simulink model "Control_try_final_2020b"  (R2020b)
settings: Solver=VariableStepAuto  StartTime=0.0  StopTime=inf  RelTol=1e-3
undefined symbols (not defined in the file or in its folder): DiscIntNeverNeededParam
libraries: mobileRoboticsLib x25
(part 6 of 7)

== stateflow chart Control_try_final_2020b/Team_1_behaviour/T1R2 (attacker 1)/Team 1 Behaviour1/kick_direction1/Chart2 ==
  state y_pos
    du:
    Vy = 1
  state y_neg
    du:
    Vy = -1
  (default) -> y_pos
  y_pos -> y_neg : [y > 0]
  y_neg -> y_pos : [y<1]
  data: y input; Vy output

== matlab function Control_try_final_2020b/Team_1_behaviour/T1R2 (attacker 1)/Team 1 Behaviour1/min_Distance_Finder/MATLAB Function ==
  data: min input; y output; rob3 input
function y = fcn(min, rob3)
 if min == rob3
y = 3;
 else 
     y =4;
 end
end

== stateflow chart Control_try_final_2020b/Team_1_behaviour/T1R2 (attacker 1)/Team 1 Behaviour1/min_Distance_Finder/R2_O_dist_val/Chart ==
  state calculate
    en:
    dist = 0;
    pos_x = 0;
    pos_y =0;
    dist_x =0;
    dist_y = 0;
    i=0;
    du:
    dist = 0;
    for i=1:7
    if (sen_1_val(i,3) > 4)
    pos_x = R_1_loc(1) + sen_1_val(i,1);
    pos_y = R_1_loc(2) + sen_1_val(i,2);
    dist_x = R_2_loc(1) - pos_x;
    dist_y = R_2_loc(2) - pos_y;
    dist = dist + sqrt((dist_x*dist_x) + (dist_y*dist_y));
    end
    end
  (default) -> calculate
  data: R_1_loc input; sen_1_val input; dist output; R_2_loc input; dist_y local; i local; pos_x local; pos_y local; dist_x local

== stateflow chart Control_try_final_2020b/Team_1_behaviour/T1R2 (attacker 1)/Team 1 Behaviour1/min_Distance_Finder/R3_O_dist_val/Chart ==
  state calculate
    en:
    dist = 0;
    pos_x = 0;
    pos_y =0;
    dist_x =0;
    dist_y = 0;
    i=0;
    du:
    dist = 0;
    for i=1:7
    if (sen_1_val(i,3) > 4)
    pos_x = R_1_loc(1) + sen_1_val(i,1);
    pos_y = R_1_loc(2) + sen_1_val(i,2);
    dist_x = R_2_loc(1) - pos_x;
    dist_y = R_2_loc(2) - pos_y;
    dist = dist + sqrt((dist_x*dist_x) + (dist_y*dist_y));
    end
    end
  (default) -> calculate
  data: R_1_loc input; sen_1_val input; dist output; R_2_loc input; dist_y local; i local; pos_x local; pos_y local; dist_x local

== stateflow chart Control_try_final_2020b/Team_1_behaviour/T1R2 (attacker 1)/Team 1 Behaviour1/min_Distance_Finder/R4_O_dist_val/Chart ==
  state calculate
    en:
    dist = 0;
    pos_x = 0;
    pos_y =0;
    dist_x =0;
    dist_y = 0;
    i=0;
    du:
    dist = 0;
    for i=1:7
    if (sen_1_val(i,3) > 4)
    pos_x = R_1_loc(1) + sen_1_val(i,1);
    pos_y = R_1_loc(2) + sen_1_val(i,2);
    dist_x = R_2_loc(1) - pos_x;
    dist_y = R_2_loc(2) - pos_y;
    dist = dist + sqrt((dist_x*dist_x) + (dist_y*dist_y));
    end
    end
  (default) -> calculate
  data: R_1_loc input; sen_1_val input; dist output; R_2_loc input; dist_y local; i local; pos_x local; pos_y local; dist_x local

== matlab function Control_try_final_2020b/Team_1_behaviour/T1R2 (attacker 1)/Team 1 Behaviour1/min_Distance_Finder/zero_padding ==
  data: u input; y output
function y = pad(u)
% Zero-pads object detections to work with arrays of buses

y = zeros(7,3);
numElems = min(size(u,1),7);
for idx = 1:numElems
   y(idx,1:3) = u(idx,1:3); 
end
end

== matlab function Control_try_final_2020b/Team_1_behaviour/T1R2 (attacker 1)/Team 1 Behaviour1/MATLAB Function3 ==
  data: distance_to_goal1 input; centroid output; goal_keeperY input; distance_to_goal2 input
function centroid  = shooting_spot_rev1_controller(distance_to_goal1, goal_keeperY, distance_to_goal2)
%UNTITLED3 Summary of this function goes here
%   Detailed explanation goes here
ShootingSpotFuzzyFile= getFISCodeGenerationData('shooting_spot_rev1');
C = evalfis(ShootingSpotFuzzyFile,[distance_to_goal1, goal_keeperY, distance_to_goal2]);
if ( C<1 )
% shooting_region=1;
centroid = [10,4.65];
elseif ( 1<=C && C<2 )
% shooting_region=2;
centroid = [10,3.35];
elseif ( 2<=C && C<3 )
% shooting_region=3;
centroid = [10,4.65];
else
% shooting_region=4;
centroid = [10,4.65];
end
end

== matlab function Control_try_final_2020b/Team_1_behaviour/T1R2 (attacker 1)/Team 1 Behaviour1/MATLAB Function2 ==
  data: u input; y output; r3 input; r4 input
function y = fcn(u , r3, r4)
if u == 3
   y = [r3(1), r3(2)];
else
    y = [r4(1) , r4(2)];
end

== matlab function Control_try_final_2020b/Team_1_behaviour/T1R2 (attacker 1)/Team 1 Behaviour1/MATLAB Function4 ==
  data: u input; y output
function y = fcn(u)
if u == 3
    y =1;
else 
    y = 0;
end
end

== matlab function Control_try_final_2020b/Team_1_behaviour/T1R3 (Defender 2)/Team 1 Behaviour1/MATLAB Function3 ==
  data: distance_to_goal1 input; centroid output; goal_keeperY input; distance_to_goal2 input
function centroid  = shooting_spot_rev1_controller(distance_to_goal1, goal_keeperY, distance_to_goal2)
%UNTITLED3 Summary of this function goes here
%   Detailed explanation goes here
ShootingSpotFuzzyFile= getFISCodeGenerationData('shooting_spot_rev1');
C = evalfis(ShootingSpotFuzzyFile,[distance_to_goal1, goal_keeperY, distance_to_goal2]);
if ( C<1 )
% shooting_region=1;
centroid = [10,4.65];
elseif ( 1<=C && C<2 )
% shooting_region=2;
centroid = [10,3.35];
elseif ( 2<=C && C<3 )
% shooting_region=3;
centroid = [10,4.65];
else
% shooting_region=4;
centroid = [10,4.65];
end
end

== matlab function Control_try_final_2020b/Team_1_behaviour/T1R3 (Defender 2)/Team 1 Behaviour1/MATLAB Function4 ==
  data: u input; y output
function y = fcn(u)
if u == 3
    y =1;
else 
    y = 0;
end
end

== stateflow chart Control_try_final_2020b/Team_1_behaviour/T1R3 (Defender 2)/Team 1 Behaviour1/kick_direction1/Chart1 ==
  state x_pos
    du:
    Vx = 1
  state x_neg
    du:
    Vx = -1
  (default) -> x_pos
  x_pos -> x_neg : [x > 0]
  x_neg -> x_pos : [x<1]
  data: Vx output; x input

== stateflow chart Control_try_final_2020b/Team_1_behaviour/T1R3 (Defender 2)/Team 1 Behaviour1/kick_direction1/Chart2 ==
  state y_pos
    du:
    Vy = 1
  state y_neg
    du:
    Vy = -1
  (default) -> y_pos
  y_pos -> y_neg : [y > 0]
  y_neg -> y_pos : [y<1]
  data: y input; Vy output

== matlab function Control_try_final_2020b/Team_1_behaviour/T1R3 (Defender 2)/Team 1 Behaviour1/min_Distance_Finder/MATLAB Function ==
  data: min input; y output; rob3 input
function y = fcn(min, rob3)
 if min == rob3
y = 3;
 else 
     y =2;
 end
end

== stateflow chart Control_try_final_2020b/Team_1_behaviour/T1R3 (Defender 2)/Team 1 Behaviour1/min_Distance_Finder/R2_O_dist_val/Chart ==
  state calculate
    en:
    dist = 0;
    pos_x = 0;
    pos_y =0;
    dist_x =0;
    dist_y = 0;
    i=0;
    du:
    dist = 0;
    for i=1:7
    if (sen_1_val(i,3) > 4)
    pos_x = R_1_loc(1) + sen_1_val(i,1);
    pos_y = R_1_loc(2) + sen_1_val(i,2);
    dist_x = R_2_loc(1) - pos_x;
    dist_y = R_2_loc(2) - pos_y;
    dist = dist + sqrt((dist_x*dist_x) + (dist_y*dist_y));
    end
    end
  (default) -> calculate
  data: R_1_loc input; sen_1_val input; dist output; R_2_loc input; dist_y local; i local; pos_x local; pos_y local; dist_x local

== stateflow chart Control_try_final_2020b/Team_1_behaviour/T1R3 (Defender 2)/Team 1 Behaviour1/min_Distance_Finder/R3_O_dist_val/Chart ==
  state calculate
    en:
    dist = 0;
    pos_x = 0;
    pos_y =0;
    dist_x =0;
    dist_y = 0;
    i=0;
    du:
    dist = 0;
    for i=1:7
    if (sen_1_val(i,3) > 4)
    pos_x = R_1_loc(1) + sen_1_val(i,1);
    pos_y = R_1_loc(2) + sen_1_val(i,2);
    dist_x = R_2_loc(1) - pos_x;
    dist_y = R_2_loc(2) - pos_y;
    dist = dist + sqrt((dist_x*dist_x) + (dist_y*dist_y));
    end
    end
  (default) -> calculate
  data: R_1_loc input; sen_1_val input; dist output; R_2_loc input; dist_y local; i local; pos_x local; pos_y local; dist_x local

== stateflow chart Control_try_final_2020b/Team_1_behaviour/T1R3 (Defender 2)/Team 1 Behaviour1/min_Distance_Finder/R4_O_dist_val/Chart ==
  state calculate
    en:
    dist = 0;
    pos_x = 0;
    pos_y =0;
    dist_x =0;
    dist_y = 0;
    i=0;
    du:
    dist = 0;
    for i=1:7
    if (sen_1_val(i,3) > 4)
    pos_x = R_1_loc(1) + sen_1_val(i,1);
    pos_y = R_1_loc(2) + sen_1_val(i,2);
    dist_x = R_2_loc(1) - pos_x;
    dist_y = R_2_loc(2) - pos_y;
    dist = dist + sqrt((dist_x*dist_x) + (dist_y*dist_y));
    end
    end
  (default) -> calculate
  data: R_1_loc input; sen_1_val input; dist output; R_2_loc input; dist_y local; i local; pos_x local; pos_y local; dist_x local

== matlab function Control_try_final_2020b/Team_2_Behaviour/T2_R3(Attacker 1)/Team 1 Behaviour1/MATLAB Function2 ==
  data: F input; dF output; dis input; dT input
function dF = fcn(F,dis,dT)


F_x_max = max(abs(F(:,1))) ;
% F_y_max = max(abs(F(:,2))) ;

Fmax = sqrt((F_x_max^2)) ;

fc = sqrt(2*dis*dis*dT) ;

if fc <= Fmax
    dF = fc ;
else
    dF = Fmax ;
end

end

== matlab function Control_try_final_2020b/Team_1_behaviour/T1R3 (Defender 2)/Team 1 Behaviour1/min_Distance_Finder/zero_padding ==
  data: u input; y output
function y = pad(u)
% Zero-pads object detections to work with arrays of buses

y = zeros(7,3);
numElems = min(size(u,1),7);
for idx = 1:numElems
   y(idx,1:3) = u(idx,1:3); 
end
end

== matlab function Control_try_final_2020b/Team_2_Behaviour/T3_R4(Attacker 2)/Team 1 Behaviour1/MATLAB Function6 ==
  data: beh input; y output; goal input; team input; rob_loc input; rob_loc1 input; z output
function [y, z] = fcn(beh,goal,team,rob_loc,rob_loc1)
if (beh == 3)
    y = goal;
    z = [10,4];
elseif (beh == 2)
    y = 0.25;
    z = [10,4];
else
    y = team;
    z = [rob_loc1(1), rob_loc1(2)];
end

== matlab function Control_try_final_2020b/Team_2_Behaviour/T3_R4(Attacker 2)/Team 1 Behaviour1/MATLAB Function7 ==
  data: u input; y output; r3 input; r4 input
function y = fcn(u , r3, r4)
if u == 6
   y = [r3(1), r3(2)];
else
    y = [r4(1) , r4(2)];
end

== matlab function Control_try_final_2020b/Team_2_Behaviour/T3_R4(Attacker 2)/Team 1 Behaviour1/MATLAB Function8 ==
  data: distance_to_goal1 input; centroid output; goal_keeperY input; distance_to_goal2 input
function centroid  = shooting_spot_rev1_controller(distance_to_goal1, goal_keeperY, distance_to_goal2)
%UNTITLED3 Summary of this function goes here
%   Detailed explanation goes here
ShootingSpotFuzzyFile= getFISCodeGenerationData('shooting_spot_rev1');
C = evalfis(ShootingSpotFuzzyFile,[distance_to_goal1, goal_keeperY, distance_to_goal2]);
if ( C<1 )
% shooting_region=1;
centroid = [10,4.65];
elseif ( 1<=C && C<2 )
% shooting_region=2;
centroid = [10,3.35];
elseif ( 2<=C && C<3 )
% shooting_region=3;
centroid = [10,4.65];
else
% shooting_region=4;
centroid = [10,4.65];
end
end

== matlab function Control_try_final_2020b/Team_2_Behaviour/T3_R4(Attacker 2)/Team 1 Behaviour1/MATLAB Function9 ==
  data: u input; y output
function y = fcn(u)
if u == 3
    y =1;
else 
    y = 0;
end
end

== stateflow chart Control_try_final_2020b/Team_2_Behaviour/T3_R4(Attacker 2)/Team 1 Behaviour1/kick_direction2/Chart1 ==
  state x_pos
    du:
    Vx = 1
  state x_neg
    du:
    Vx = -1
  (default) -> x_pos
  x_pos -> x_neg : [x > 0]
  x_neg -> x_pos : [x<1]
  data: Vx output; x input

== stateflow chart Control_try_final_2020b/Team_2_Behaviour/T3_R4(Attacker 2)/Team 1 Behaviour1/kick_direction2/Chart2 ==
  state y_pos
    du:
    Vy = 1
  state y_neg
    du:
    Vy = -1
  (default) -> y_pos
  y_pos -> y_neg : [y > 0]
  y_neg -> y_pos : [y<1]
  data: y input; Vy output

== matlab function Control_try_final_2020b/Team_2_Behaviour/T3_R4(Attacker 2)/Team 1 Behaviour1/min_Distance_Finder1/MATLAB Function ==
  data: min input; y output; rob3 input
function y = fcn(min, rob3)
 if min == rob3
y = 6;
 else 
     y =7;
 end
end

== stateflow chart Control_try_final_2020b/Team_2_Behaviour/T3_R4(Attacker 2)/Team 1 Behaviour1/min_Distance_Finder1/R2_O_dist_val/Chart ==
  state calculate
    en:
    dist = 0;
    pos_x = 0;
    pos_y =0;
    dist_x =0;
    dist_y = 0;
    i=0;
    du:
    dist = 0;
    for i=1:7
    if (sen_1_val(i,3) > 4)
    pos_x = R_1_loc(1) + sen_1_val(i,1);
    pos_y = R_1_loc(2) + sen_1_val(i,2);
    dist_x = R_2_loc(1) - pos_x;
    dist_y = R_2_loc(2) - pos_y;
    dist = sqrt((dist_x*dist_x) + (dist_y*dist_y));
    end
    end
  (default) -> calculate
  data: R_1_loc input; sen_1_val input; dist output; R_2_loc input; dist_y local; i local; pos_x local; pos_y local; dist_x local

== stateflow chart Control_try_final_2020b/Referee/GOAL ==
  state Start
    en:
    right_team_goal = 0;
    left_team_goal = 0;
    reset = 0;
    right_team_stop = 0;
    left_team_stop = 1;
  state in_field
    du:
    reset = 0
    left_team_stop = 0;
    right_team_stop = 0;
  state Goal_right
    en:
    left_team_goal = left_team_goal + 1;
    reset = 1
    left_team_stop = 1;
  state Goal_left
    en:
    right_team_goal = right_team_goal +1;
    reset = 1
    right_team_stop = 1;
  (default) -> Start
  Start -> in_field : [X > 1 && X<10 && Y > 1  && Y < 7 && after(3, sec)]
  Goal_right -> in_field : [X > 1 && X<10 && Y > 1  && Y < 7 ]
  Goal_left -> in_field : [X > 1 && X<10 && Y > 1  && Y < 7]
  in_field -> Goal_right [order 1] : [fix(X) == 10 && Y > 2.7  && Y < 5.3 && Z <1.2]
  in_field -> Goal_left [order 2] : [round(X+0.5) == 1 && Y > 2.7  && Y < 5.3 && Z < 1.2]
  data: X input; Y input size=1; Z input; left_team_goal output; reset output; left_team_stop output; right_team_stop output; right_team_goal output

== stateflow chart Control_try_final_2020b/Team_2_Behaviour/T3_R4(Attacker 2)/Team 1 Behaviour1/min_Distance_Finder1/R3_O_dist_val/Chart ==
  state calculate
    en:
    dist = 0;
    pos_x = 0;
    pos_y =0;
    dist_x =0;
    dist_y = 0;
    i=0;
    du:
    dist = 0;
    for i=1:7
    if (sen_1_val(i,3) > 4)
    pos_x = R_1_loc(1) + sen_1_val(i,1);
    pos_y = R_1_loc(2) + sen_1_val(i,2);
    dist_x = R_2_loc(1) - pos_x;
    dist_y = R_2_loc(2) - pos_y;
    dist = dist + sqrt((dist_x*dist_x) + (dist_y*dist_y));
    end
    end
  (default) -> calculate
  data: R_1_loc input; sen_1_val input; dist output; R_2_loc input; dist_y local; i local; pos_x local; pos_y local; dist_x local

== stateflow chart Control_try_final_2020b/Team_2_Behaviour/T3_R4(Attacker 2)/Team 1 Behaviour1/min_Distance_Finder1/R4_O_dist_val/Chart ==
  state calculate
    en:
    dist = 0;
    pos_x = 0;
    pos_y =0;
    dist_x =0;
    dist_y = 0;
    i=0;
    du:
    dist = 0;
    for i=1:7
    if (sen_1_val(i,3) > 4)
    pos_x = R_1_loc(1) + sen_1_val(i,1);
    pos_y = R_1_loc(2) + sen_1_val(i,2);
    dist_x = R_2_loc(1) - pos_x;
    dist_y = R_2_loc(2) - pos_y;
    dist = dist + sqrt((dist_x*dist_x) + (dist_y*dist_y));
    end
    end
  (default) -> calculate
  data: R_1_loc input; sen_1_val input; dist output; R_2_loc input; dist_y local; i local; pos_x local; pos_y local; dist_x local

== stateflow chart Control_try_final_2020b/Team_2_Behaviour/T3_R4(Attacker 2)/Team 1 Behaviour1/min_Distance_Finder1/nearest robot distance/Chart ==
  state calculate
    en:
    dist = 0;
    pos_x = 0;
    pos_y =0;
    dist_x =0;
    dist_y = 0;
    i=0;
    du:
    dist = 0;
    for i=1:7
    if (sen_1_val(i,3) < 9)
    pos_x = R_1_loc(1) + sen_1_val(i,1);
    pos_y = R_1_loc(2) + sen_1_val(i,2);
    dist_x = R_1_loc(1) - pos_x;
    dist_y = R_1_loc(2) - pos_y;
    dist = dist + sqrt((dist_x*dist_x) + (dist_y*dist_y));
    end
    end
  (default) -> calculate
  data: R_1_loc input; sen_1_val input; dist output; dist_y local; i local; pos_x local; pos_y local; dist_x local

== matlab function Control_try_final_2020b/Team_2_Behaviour/T3_R4(Attacker 2)/Team 1 Behaviour1/min_Distance_Finder1/zero_padding ==
  data: u input; y output
function y = pad(u)
% Zero-pads object detections to work with arrays of buses

y = zeros(7,3);
numElems = min(size(u,1),7);
for idx = 1:numElems
   y(idx,1:3) = u(idx,1:3); 
end
end

== matlab function Control_try_final_2020b/Team_2_Behaviour/T2_R2(defender)/Team 1 Behaviour1/MATLAB Function2 ==
  data: u input; y output; r3 input; r4 input
function y = fcn(u , r3, r4)
if u == 8
   y = [r3(1), r3(2)];
else
    y = [r4(1) , r4(2)];
end

== matlab function Control_try_final_2020b/Team_2_Behaviour/T2_R2(defender)/Team 1 Behaviour1/MATLAB Function3 ==
  data: distance_to_goal1 input; centroid output; goal_keeperY input; distance_to_goal2 input
function centroid  = shooting_spot_rev1_controller(distance_to_goal1, goal_keeperY, distance_to_goal2)
%UNTITLED3 Summary of this function goes here
%   Detailed explanation goes here
ShootingSpotFuzzyFile= getFISCodeGenerationData('shooting_spot_rev1');
C = evalfis(ShootingSpotFuzzyFile,[distance_to_goal1, goal_keeperY, distance_to_goal2]);
if ( C<1 )
% shooting_region=1;
centroid = [10,4.65];
elseif ( 1<=C && C<2 )
% shooting_region=2;
centroid = [10,3.35];
elseif ( 2<=C && C<3 )
% shooting_region=3;
centroid = [10,4.65];
else
% shooting_region=4;
centroid = [10,4.65];
end
end

== matlab function Control_try_final_2020b/Team_2_Behaviour/T2_R2(defender)/Team 1 Behaviour1/MATLAB Function4 ==
  data: u input; y output
function y = fcn(u)
if u == 3
    y =1;
else 
    y = 0;
end
end

== stateflow chart Control_try_final_2020b/Team_2_Behaviour/T2_R2(defender)/Team 1 Behaviour1/kick_direction1/Chart1 ==
  state x_pos
    du:
    Vx = 1
  state x_neg
    du:
    Vx = -1
  (default) -> x_pos
  x_pos -> x_neg : [x > 0]
  x_neg -> x_pos : [x<1]
  data: Vx output; x input

== stateflow chart Control_try_final_2020b/Team_2_Behaviour/T2_R2(defender)/Team 1 Behaviour1/kick_direction1/Chart2 ==
  state y_pos
    du:
    Vy = 1
  state y_neg
    du:
    Vy = -1
  (default) -> y_pos
  y_pos -> y_neg : [y > 0]
  y_neg -> y_pos : [y<1]
  data: y input; Vy output

== matlab function Control_try_final_2020b/Team_2_Behaviour/T2_R2(defender)/Team 1 Behaviour1/min_Distance_Finder/MATLAB Function ==
  data: min input; y output; rob3 input
function y = fcn(min, rob3)
 if min == rob3
y = 8;
 else 
     y =7;
 end
end

== stateflow chart Control_try_final_2020b/Team_2_Behaviour/T2_R2(defender)/Team 1 Behaviour1/min_Distance_Finder/R2_O_dist_val/Chart ==
  state calculate
    en:
    dist = 0;
    pos_x = 0;
    pos_y =0;
    dist_x =0;
    dist_y = 0;
    i=0;
    du:
    dist = 0;
    for i=1:7
    if (sen_1_val(i,3) > 4)
    pos_x = R_1_loc(1) + sen_1_val(i,1);
    pos_y = R_1_loc(2) + sen_1_val(i,2);
    dist_x = R_2_loc(1) - pos_x;
    dist_y = R_2_loc(2) - pos_y;
    dist = sqrt((dist_x*dist_x) + (dist_y*dist_y));
    end
    end
  (default) -> calculate
  data: R_1_loc input; sen_1_val input; dist output; R_2_loc input; dist_y local; i local; pos_x local; pos_y local; dist_x local

== stateflow chart Control_try_final_2020b/Team_2_Behaviour/T2_R2(defender)/Team 1 Behaviour1/min_Distance_Finder/R3_O_dist_val/Chart ==
  state calculate
    en:
    dist = 0;
    pos_x = 0;
    pos_y =0;
    dist_x =0;
    dist_y = 0;
    i=0;
    du:
    dist = 0;
    for i=1:7
    if (sen_1_val(i,3) > 4)
    pos_x = R_1_loc(1) + sen_1_val(i,1);
    pos_y = R_1_loc(2) + sen_1_val(i,2);
    dist_x = R_2_loc(1) - pos_x;
    dist_y = R_2_loc(2) - pos_y;
    dist = dist + sqrt((dist_x*dist_x) + (dist_y*dist_y));
    end
    end
  (default) -> calculate
  data: R_1_loc input; sen_1_val input; dist output; R_2_loc input; dist_y local; i local; pos_x local; pos_y local; dist_x local

== stateflow chart Control_try_final_2020b/Team_2_Behaviour/T2_R2(defender)/Team 1 Behaviour1/min_Distance_Finder/R4_O_dist_val/Chart ==
  state calculate
    en:
    dist = 0;
    pos_x = 0;
    pos_y =0;
    dist_x =0;
    dist_y = 0;
    i=0;
    du:
    dist = 0;
    for i=1:7
    if (sen_1_val(i,3) > 4)
    pos_x = R_1_loc(1) + sen_1_val(i,1);
    pos_y = R_1_loc(2) + sen_1_val(i,2);
    dist_x = R_2_loc(1) - pos_x;
    dist_y = R_2_loc(2) - pos_y;
    dist = dist + sqrt((dist_x*dist_x) + (dist_y*dist_y));
    end
    end
  (default) -> calculate
  data: R_1_loc input; sen_1_val input; dist output; R_2_loc input; dist_y local; i local; pos_x local; pos_y local; dist_x local

== stateflow chart Control_try_final_2020b/Team_2_Behaviour/T2_R2(defender)/Team 1 Behaviour1/min_Distance_Finder/nearest robot distance/Chart ==
  state calculate
    en:
    dist = 0;
    pos_x = 0;
    pos_y =0;
    dist_x =0;
    dist_y = 0;
    i=0;
    du:
    dist = 0;
    for i=1:7
    if (sen_1_val(i,3) < 9)
    pos_x = R_1_loc(1) + sen_1_val(i,1);
    pos_y = R_1_loc(2) + sen_1_val(i,2);
    dist_x = R_1_loc(1) - pos_x;
    dist_y = R_1_loc(2) - pos_y;
    dist = dist + sqrt((dist_x*dist_x) + (dist_y*dist_y));
    end
    end
  (default) -> calculate
  data: R_1_loc input; sen_1_val input; dist output; dist_y local; i local; pos_x local; pos_y local; dist_x local

== matlab function Control_try_final_2020b/Team_2_Behaviour/T2_R2(defender)/Team 1 Behaviour1/min_Distance_Finder/zero_padding ==
  data: u input; y output
function y = pad(u)
% Zero-pads object detections to work with arrays of buses

y = zeros(7,3);
numElems = min(size(u,1),7);
for idx = 1:numElems
   y(idx,1:3) = u(idx,1:3); 
end
end

== matlab function Control_try_final_2020b/Team_2_Behaviour/T2_R3(Attacker 1)/Team 1 Behaviour1/MATLAB Function4 ==
  data: u input; y output; r3 input; r4 input
function y = fcn(u , r3, r4)
if u == 6
   y = [r3(1), r3(2)];
else
    y = [r4(1) , r4(2)];
end

== matlab function Control_try_final_2020b/Team_2_Behaviour/T2_R3(Attacker 1)/Team 1 Behaviour1/MATLAB Function5 ==
  data: distance_to_goal1 input; centroid output; goal_keeperY input; distance_to_goal2 input
function centroid  = shooting_spot_rev1_controller(distance_to_goal1, goal_keeperY, distance_to_goal2)
%UNTITLED3 Summary of this function goes here
%   Detailed explanation goes here
ShootingSpotFuzzyFile= getFISCodeGenerationData('shooting_spot_rev1');
C = evalfis(ShootingSpotFuzzyFile,[distance_to_goal1, goal_keeperY, distance_to_goal2]);
if ( C<1 )
% shooting_region=1;
centroid = [10,4.65];
elseif ( 1<=C && C<2 )
% shooting_region=2;
centroid = [10,3.35];
elseif ( 2<=C && C<3 )
% shooting_region=3;
centroid = [10,4.65];
else
% shooting_region=4;
centroid = [10,4.65];
end
end

== matlab function Control_try_final_2020b/Team_2_Behaviour/T2_R3(Attacker 1)/Team 1 Behaviour1/MATLAB Function6 ==
  data: u input; y output
function y = fcn(u)
if u == 3
    y =1;
else 
    y = 0;
end
end

== stateflow chart Control_try_final_2020b/Team_2_Behaviour/T2_R3(Attacker 1)/Team 1 Behaviour1/kick_direction1/Chart1 ==
  state x_pos
    du:
    Vx = 1
  state x_neg
    du:
    Vx = -1
  (default) -> x_pos
  x_pos -> x_neg : [x > 0]
  x_neg -> x_pos : [x<1]
  data: Vx output; x input

== stateflow chart Control_try_final_2020b/Team_2_Behaviour/T2_R3(Attacker 1)/Team 1 Behaviour1/kick_direction1/Chart2 ==
  state y_pos
    du:
    Vy = 1
  state y_neg
    du:
    Vy = -1
  (default) -> y_pos
  y_pos -> y_neg : [y > 0]
  y_neg -> y_pos : [y<1]
  data: y input; Vy output

== matlab function Control_try_final_2020b/Team_2_Behaviour/T2_R3(Attacker 1)/Team 1 Behaviour1/MATLAB Function3 ==
  data: beh input; y output; goal input; team input; rob_loc input; rob_loc1 input; z output
function [y, z] = fcn(beh,goal,team,rob_loc,rob_loc1)
if (beh == 3)
    y = goal;
    z = [10,4];
elseif (beh == 2)
    y = 0.25;
    z = [10,4];
else
    y = team;
    z = [rob_loc1(1), rob_loc1(2)];
end

== matlab function Control_try_final_2020b/Team_2_Behaviour/T2_R3(Attacker 1)/Team 1 Behaviour1/min_Distance_Finder1/MATLAB Function ==
  data: min input; y output; rob3 input
function y = fcn(min, rob3)
 if min == rob3
y = 6;
 else 
     y =8;
 end
end

== stateflow chart Control_try_final_2020b/Team_2_Behaviour/T2_R3(Attacker 1)/Team 1 Behaviour1/min_Distance_Finder1/R2_O_dist_val/Chart ==
  state calculate
    en:
    dist = 0;
    pos_x = 0;
    pos_y =0;
    dist_x =0;
    dist_y = 0;
    i=0;
    du:
    dist = 0;
    for i=1:7
    if (sen_1_val(i,3) > 4)
    pos_x = R_1_loc(1) + sen_1_val(i,1);
    pos_y = R_1_loc(2) + sen_1_val(i,2);
    dist_x = R_2_loc(1) - pos_x;
    dist_y = R_2_loc(2) - pos_y;
    dist = sqrt((dist_x*dist_x) + (dist_y*dist_y));
    end
    end
  (default) -> calculate
  data: R_1_loc input; sen_1_val input; dist output; R_2_loc input; dist_y local; i local; pos_x local; pos_y local; dist_x local

== stateflow chart Control_try_final_2020b/Team_2_Behaviour/T2_R3(Attacker 1)/Team 1 Behaviour1/min_Distance_Finder1/R3_O_dist_val/Chart ==
  state calculate
    en:
    dist = 0;
    pos_x = 0;
    pos_y =0;
    dist_x =0;
    dist_y = 0;
    i=0;
    du:
    dist = 0;
    for i=1:7
    if (sen_1_val(i,3) > 4)
    pos_x = R_1_loc(1) + sen_1_val(i,1);
    pos_y = R_1_loc(2) + sen_1_val(i,2);
    dist_x = R_2_loc(1) - pos_x;
    dist_y = R_2_loc(2) - pos_y;
    dist = dist + sqrt((dist_x*dist_x) + (dist_y*dist_y));
    end
    end
  (default) -> calculate
  data: R_1_loc input; sen_1_val input; dist output; R_2_loc input; dist_y local; i local; pos_x local; pos_y local; dist_x local

== stateflow chart Control_try_final_2020b/Team_2_Behaviour/T2_R3(Attacker 1)/Team 1 Behaviour1/min_Distance_Finder1/R4_O_dist_val/Chart ==
  state calculate
    en:
    dist = 0;
    pos_x = 0;
    pos_y =0;
    dist_x =0;
    dist_y = 0;
    i=0;
    du:
    dist = 0;
    for i=1:7
    if (sen_1_val(i,3) > 4)
    pos_x = R_1_loc(1) + sen_1_val(i,1);
    pos_y = R_1_loc(2) + sen_1_val(i,2);
    dist_x = R_2_loc(1) - pos_x;
    dist_y = R_2_loc(2) - pos_y;
    dist = dist + sqrt((dist_x*dist_x) + (dist_y*dist_y));
    end
    end
  (default) -> calculate
  data: R_1_loc input; sen_1_val input; dist output; R_2_loc input; dist_y local; i local; pos_x local; pos_y local; dist_x local

== stateflow chart Control_try_final_2020b/Team_2_Behaviour/T2_R3(Attacker 1)/Team 1 Behaviour1/min_Distance_Finder1/nearest robot distance/Chart ==
  state calculate
    en:
    dist = 0;
    pos_x = 0;
    pos_y =0;
    dist_x =0;
    dist_y = 0;
    i=0;
    du:
    dist = 0;
    for i=1:7
    if (sen_1_val(i,3) < 9)
    pos_x = R_1_loc(1) + sen_1_val(i,1);
    pos_y = R_1_loc(2) + sen_1_val(i,2);
    dist_x = R_1_loc(1) - pos_x;
    dist_y = R_1_loc(2) - pos_y;
    dist = dist + sqrt((dist_x*dist_x) + (dist_y*dist_y));
    end
    end
  (default) -> calculate
  data: R_1_loc input; sen_1_val input; dist output; dist_y local; i local; pos_x local; pos_y local; dist_x local

== matlab function Control_try_final_2020b/Team_2_Behaviour/T2_R3(Attacker 1)/Team 1 Behaviour1/min_Distance_Finder1/zero_padding ==
  data: u input; y output
function y = pad(u)
% Zero-pads object detections to work with arrays of buses

y = zeros(7,3);
numElems = min(size(u,1),7);
for idx = 1:numElems
   y(idx,1:3) = u(idx,1:3); 
end
end

== stateflow chart Control_try_final_2020b/Referee/Corner ==
  state Start
    en:
    CFR = 0;
    CFL = 0;
    C_foul_loc = [0;0]
  state foul_left
    en:
    if (ball_tag<5)
    CFL = 1;
    if (Y < 4)
    C_foul_loc  = [1;1]
    elseif (Y>4)
    C_foul_loc  = [1;7]
    end
    else
    CFR = 1;
    C_foul_loc  = [1.5;4]
    end
  state foul_right
    en:
    if (ball_tag>4)
    CFR = 1;
    C_foul_loc  = [10;4]
    else
    CFL =2;
    if (Y<1)
    C_foul_loc  = [10;1]
    elseif (Y>7)
    C_foul_loc  = [10;7]
    end
    end
  state in_field
    en:
    CFR = 0;
    CFL = 0;
  (default) -> Start
  Start -> in_field
  foul_right -> in_field : [ X> 1  && X< 10]
  foul_left -> in_field : [X> 1  && X< 10]
  in_field -> foul_left [order 2] : [X < 1 && (Y < 2.7 || Y > 5.3)]
  in_field -> foul_right [order 1] : [X > 10 && (Y < 2.7 || Y > 5.3)]
  data: ball_tag input; X input; Y input; CFR output; CFL output; C_foul_loc output

== stateflow chart Control_try_final_2020b/Referee/Chart ==
  state Start
    en:
    dist= 0;
    flag=0;
    team_bot1 =0;
    team_bot2 =0;
  state collision_detector
    en:
    team_bot1 =0;
    team_bot2 =0;
    i=0
    j=0
    du:
    for i=1:4
    for j=1:4
    dist=sqrt((bot_loc_arr(1,i)-bot_loc_arr(1,j+4))^2+(bot_loc_arr(2,i)-bot_loc_arr(2,j+4))^2)
    if (dist<0.25)
    flag=1;
    team_bot1=i;
    team_bot2=j+4;
    break
    end
    end
    if flag==1
    break
    end
    end
  state foul_detector
    en:
    if (bot_vel(team_bot1) > bot_vel(team_bot2))
    col_team_1 = 1;
    col_team_2 = 0;
    else
    col_team_1 = 0;
    col_team_2 = 1;
    end
    col_ball_loc = team_bot1;
    flag = 0;
  (default) -> Start
  Start -> collision_detector
  foul_detector -> collision_detector : [ flag==0 && after(5,sec)]
  collision_detector -> foul_detector : [flag==1]
  data: bot_vel input; bot_loc_arr input; col_ball_loc output; dist local; flag local; i local; j local; col_team_1 output; col_team_2 output; team_bot1 local; team_bot2 local

== matlab function Control_try_final_2020b/Enviornment/MATLAB Function ==

function plotEnvironment

coder.extrinsic('evalin');
persistent hasPlotted
if isempty(hasPlotted)
    evalin('base','environment_Plot');
    hasPlotted = true;
end

== stateflow chart Control_try_final_2020b/Enviornment/Ball_Dynamics/Chart ==
  state on_ground
    du:
    if(abs(F)>2.6)
    a = (abs(F)-2.6) * (F/abs(F)) / 0.43
    else
    a = 0
    end
  state off_ground
    du:
    a = F/0.43
  (default) -> on_ground
  off_ground -> on_ground : [Y ==0]
  on_ground -> off_ground : [Y > 0]
  data: Y input; F input; a output

== stateflow chart Control_try_final_2020b/Enviornment/Ball_Dynamics/Chart1 ==
  state calculations_neg
    du:
    vs = (abs(v))*(abs(v))*(-1)
  state calculations_pos
    du:
    vs = v*v
  (default) -> calculations_neg
  calculations_pos -> calculations_neg : [v<0]
  calculations_neg -> calculations_pos : [v>0]
  data: vs output; v input

== stateflow chart Control_try_final_2020b/Enviornment/Ball_Dynamics/Chart2 ==
  state on_ground
    du:
    if(abs(F)>2.6)
    a = (abs(F) - 2.6) * (F/abs(F)) / 0.43
    else
    a = 0
    end
  state off_ground
    du:
    a = F/0.43
  (default) -> on_ground
  off_ground -> on_ground : [Y ==0]
  on_ground -> off_ground : [Y > 0]
  data: Y input; F input; a output

== stateflow chart Control_try_final_2020b/Enviornment/Ball_Dynamics/Chart3 ==
  state calculations_neg
    du:
    vs = (abs(v))*(abs(v))*(-1)
  state calculations_pos
    du:
    vs = v*v
  (default) -> calculations_neg
  calculations_pos -> calculations_neg : [v<0]
  calculations_neg -> calculations_pos : [v>=0]
  data: vs output; v input

== stateflow chart Control_try_final_2020b/Enviornment/Ball_Dynamics/Chart4 ==
  state in_motion
    du:
    if (v > 0)
    a = -(0.32*0.98)
    else if(v<0)
    a = (0.32*0.98)
    end
    end
  state stationary
    du:
    a = 0;
  (default) -> in_motion
  in_motion -> stationary : [abs(v) < 0.03 | Y>0]
  stationary -> in_motion : [abs(v)>0.03]
  data: Y input; a output; v input

== stateflow chart Control_try_final_2020b/Team_1_behaviour/T1R1(Goal_Keeper)/Chart ==
  state in_D
    du:
    D = 0
  state out_D
    du:
    D=1
  (default) -> in_D
  in_D -> out_D : [ X<1.1 || X>2.5 || Y<2.7 || Y>5.3]
  out_D -> in_D : [X>1.1 && X<2.5 && Y>2.7 && Y<5.3]
  data: X input; Y input; D output

== stateflow chart Control_try_final_2020b/Enviornment/Ball_Dynamics/Chart6 ==
  state in_motion
    du:
    if (v > 0)
    a = -(0.32*0.98)
    else if(v<0)
    a = (0.32*0.98)
    end
    end
  state stationary
    du:
    a = 0;
  (default) -> in_motion
  in_motion -> stationary : [abs(v) < 0.01 | Y>0]
  stationary -> in_motion : [abs(v)>0.02]
  data: Y input; a output; v input

== stateflow chart Control_try_final_2020b/Team_1_behaviour/T1R1(Goal_Keeper)/ball_out_of_D/control ==
  state Ball_Following_ball_out_D
    du:
    kick = 0;
    if (R1_loc_Y>2.7 && R1_loc_Y<5.3)
    if(Ball_loc_Y > R1_loc_Y)
    R1_vel_Y = 0.1;
    elseif (Ball_loc_Y < R1_loc_Y)
    R1_vel_Y = -0.1;
    end
    elseif ( R1_loc_Y > 5.3)
    R1_vel_Y = -0.1;
    elseif ( R1_loc_Y < 2.7)
    R1_vel_Y = 0.1;
    end
    end
  state Ball_Held
    du:
    kick = 1;
  (default) -> Ball_Following_ball_out_D
  Ball_Following_ball_out_D -> Ball_Held : [GB_dist < 0.25]
  Ball_Held -> Ball_Following_ball_out_D : [GB_dist > 0.25]
  data: kick output; R1_loc_X input; Ball_loc_X input; GB_dist input; R1_loc_Y input; Ball_loc_Y input; R1_vel_Y output

== stateflow chart Control_try_final_2020b/Team_1_behaviour/T1R3 (Defender 2)/Team 1 Behaviour1/Chart1 ==
  state second_coordinate
    du:
    actual_angle = -pi +angle + angle_bot;
  state first_coordinate
    du:
    actual_angle = angle_bot - angle;
  state ffourth_coordinate
    du:
    actual_angle = -(2*pi) + angle + angle_bot
  state Third_coordinate
    du:
    actual_angle =-(pi) - angle + angle_bot;
  (default) -> first_coordinate
  first_coordinate -> second_coordinate [order 1] : [ Rx>Bx && Ry<By ]
  second_coordinate -> first_coordinate [order 1] : [ Rx<Bx && Ry<By]
  ffourth_coordinate -> second_coordinate [order 1] : [ Rx>Bx && Ry<By ]
  first_coordinate -> Third_coordinate [order 3] : [ Rx>Bx && Ry>By]
  second_coordinate -> Third_coordinate [order 3] : [ Rx>Bx && Ry>By ]
  Third_coordinate -> second_coordinate [order 1] : [ Rx>Bx && Ry<By ]
  second_coordinate -> ffourth_coordinate [order 2] : [ Rx<Bx && Ry>By ]
  Third_coordinate -> first_coordinate [order 2] : [ Rx<Bx && Ry<By ]
  ffourth_coordinate -> first_coordinate [order 2] : [ Rx<Bx && Ry<By ]
  first_coordinate -> ffourth_coordinate [order 2] : [ Rx<Bx && Ry>By ]
  Third_coordinate -> ffourth_coordinate [order 3] : [ Rx<Bx && Ry>By ]
  ffourth_coordinate -> Third_coordinate [order 3] : [ Rx>Bx && Ry>By]
  data: Bx input; By input; Rx input; Ry input; angle input; actual_angle output; angle_bot input

== stateflow chart Control_try_final_2020b/Team_1_behaviour/T1R3 (defender 1)/Chart ==
  state reaching_foul
    du:
    velocity_UA = 1;
    dest = [bx;by;0];
  state ball_in_other_half_did_foul
    en:
    if (foul_loc_y>=7)
    dest = [foul_loc_x;foul_loc_y - 1;0];
    elseif(foul_loc_y<=1)
    dest = [foul_loc_x;foul_loc_y + 1;0];
    end
    kick_UA = 1;
    stop = 1;
  state throwing_foul_not_done
    du:
    [foul_loc_x;foul_loc_y;0];
    kick_UA = 1;
  state stop_bot1
    du:
    velocity_UA = 1;
    dest = [bx;by;0];
  state dont_stop_bot1
    du:
    velocity_UA = 1;
    dest = [bx;by;0];
  state throwing_foul_done
    du:
  state ball_in_our_half
    en:
    dest = [3.25;5.5;0];
    kick_UA = 1;
  state init_pos_reached2
    du:
    velocity_UA = 1;
    dest = [bx;by;0];
  state in_play
    du:
    dest = [bx;by;0];
    kick_UA = 0;
    stop = 0
    velocity_UA = 0;
  state goal1
    en:
    dest = [3.25;5.5;0];
    kick_UA = 1;
    if (did_goal == 1)
    stop = 1;
    else
    stop = 0;
    end
  state init_pos_reached1
    du:
  throwing_foul_not_done -> ball_in_our_half [order 2] : [foul_loc_x > 5.5]
  ball_in_other_half_did_foul -> reaching_foul : [R_2_loc(1) < foul_loc_x + 0.25 &&  R_2_loc(1) > foul_loc_x- 0.25 && R_2_loc(2) < foul_loc_y + 1.25 &&  R_2_loc(2) > foul_loc_y - 1.25 && after(3,sec)]
  reaching_foul -> in_play : [bx >foul_loc_x + 0.1  || bx < foul_loc_x - 0.1|| by >foul_loc_y + 0.1 || by<foul_loc_y - 0.1]
  init_pos_reached1 -> dont_stop_bot1 [order 2] : [stop == 0]
  throwing_foul_done -> ball_in_other_half_did_foul [order 1] : [foul_loc_x < 5.5]
  in_play -> throwing_foul_not_done [order 3] : [foul_team_right == 1 && after(1,sec)]
  throwing_foul_not_done -> in_play [order 1] : [foul_loc_x < 5.5 && after(20,sec) &&  bx < foul_loc_x + 0.1  && bx > foul_loc_x - 0.1 && by < foul_loc_y + 0.1  && by > foul_loc_y - 0.1]
  init_pos_reached1 -> stop_bot1 [order 1] : [stop == 1]
  throwing_foul_done -> ball_in_our_half [order 2] : [foul_loc_x > 5.5]
  in_play -> throwing_foul_done [order 1] : [foul_team_left == 1]
  dont_stop_bot1 -> in_play : [reset == 0 && after(3,sec)]
  stop_bot1 -> in_play : [bx > 5.6 || bx < 5.4 || by >4.1 || by<3.9]
  ball_in_our_half -> init_pos_reached2 : [R_2_loc(1) <3.5 &&  R_2_loc(1) >3 && R_2_loc(2) <5.75 &&  R_2_loc(2) >5.25 && after(3,sec) ]
  (default) -> in_play
  goal1 -> init_pos_reached1 : [R_2_loc(1) <3.5 &&  R_2_loc(1) >3 && R_2_loc(2) <5.75 &&  R_2_loc(2) >5.25 && after(3,sec) ]
  init_pos_reached2 -> in_play : [[bx >foul_loc_x + 0.1  || bx < foul_loc_x - 0.1|| by >foul_loc_y + 0.1 || by<foul_loc_y - 0.1]]
  in_play -> goal1 [order 2] : [reset == 1]
  data: R_2_loc input; bx input; by input; foul_team_left input; foul_loc_x input; foul_loc_y input; foul_team_right input; reset input; dest output; kick_UA output; velocity_UA output; did_goal input; stop local

== stateflow chart Control_try_final_2020b/Team_1_behaviour/T1R1(Goal_Keeper)/min_Distance_Finder/Kick_prob_calc ==
  state bot_2
    du:
    kick_direction = R_2_loc
  state bot_3
    du:
    kick_direction = R_3_loc
  state bot_4
    du:
    kick_direction = R_4_loc
  (default) -> bot_2
  bot_2 -> bot_3 [order 1] : [R1_R3_dis < R1_R2_dis && R1_R3_dis < R1_R4_dis]
  bot_3 -> bot_2 [order 1] : [R1_R2_dis < R1_R3_dis && R1_R2_dis < R1_R4_dis]
  bot_4 -> bot_2 [order 2] : [R1_R2_dis < R1_R3_dis && R1_R2_dis < R1_R4_dis]
  bot_2 -> bot_4 [order 2] : [R1_R4_dis < R1_R3_dis && R1_R4_dis < R1_R2_dis]
  bot_3 -> bot_4 [order 2] : [R1_R4_dis < R1_R3_dis && R1_R4_dis < R1_R2_dis]
  bot_4 -> bot_3 [order 1] : [R1_R3_dis < R1_R2_dis && R1_R3_dis < R1_R4_dis]
  data: R_4_loc input; R_2_loc input; R_3_loc input; R1_R2_dis input; R1_R3_dis input; R1_R4_dis input; kick_direction output

== stateflow chart Control_try_final_2020b/Team_1_behaviour/T1R1(Goal_Keeper)/min_Distance_Finder/R2_O_dist_val/Chart ==
  state calculate
    en:
    dist = 0;
    pos_x = 0;
    pos_y =0;
    dist_x =0;
    dist_y = 0;
    i=0;
    du:
    dist = 0;
    for i=1:7
    if (sen_1_val(i,3) > 4)
    pos_x = R_1_loc(1) + sen_1_val(i,1);
    pos_y = R_1_loc(2) + sen_1_val(i,2);
    dist_x = R_2_loc(1) - pos_x;
    dist_y = R_2_loc(2) - pos_y;
    dist = dist + sqrt((dist_x*dist_x) + (dist_y*dist_y));
    end
    end
  (default) -> calculate
  data: R_1_loc input; sen_1_val input; dist output; R_2_loc input; dist_y local; i local; pos_x local; pos_y local; dist_x local

== stateflow chart Control_try_final_2020b/Team_1_behaviour/T1R1(Goal_Keeper)/min_Distance_Finder/R3_O_dist_val/Chart ==
  state calculate
    en:
    dist = 0;
    pos_x = 0;
    pos_y =0;
    dist_x =0;
    dist_y = 0;
    i=0;
    du:
    dist = 0;
    for i=1:7
    if (sen_1_val(i,3) > 4)
    pos_x = R_1_loc(1) + sen_1_val(i,1);
    pos_y = R_1_loc(2) + sen_1_val(i,2);
    dist_x = R_2_loc(1) - pos_x;
    dist_y = R_2_loc(2) - pos_y;
    dist = dist + sqrt((dist_x*dist_x) + (dist_y*dist_y));
    end
    end
  (default) -> calculate
  data: R_1_loc input; sen_1_val input; dist output; R_2_loc input; dist_y local; i local; pos_x local; pos_y local; dist_x local

== stateflow chart Control_try_final_2020b/Enviornment/kick_director/Chart ==
  state P1_kick
    du:
    KF = [p1(1);p1(2);p1(3);p1(4)]
    %bot_tag = 1
  state P5_kick
    du:
    KF = [p5(1);p5(2);p5(3);p5(4)]
    %KF = p5
    %bot_tag = 5
  state no_ball_kick
    du:
    KF = [0;0;0;0]
  state P2_kick
    du:
    KF = p2
    %bot_tag = 2
  state P6_kick
    du:
    KF = p6
    %bot_tag = 6
  state P3_kick
    du:
    KF = p3
    %bot_tag = 3
  state P7_kick
    du:
    KF = p7
    %bot_tag = 7
  state P4_kick
    du:
    KF = p4
    %bot_tag = 4
  state P8_kick
    du:
    KF = p8
    %bot_tag = 8
  (default) -> no_ball_kick
  P5_kick -> no_ball_kick : [p5(4) == 0]
  P1_kick -> no_ball_kick : [p1(4) == 0]
  no_ball_kick -> P5_kick [order 5] : [p5(4) == 1]
  no_ball_kick -> P1_kick [order 1] : [p1(4) == 1]
  no_ball_kick -> P2_kick [order 2] : [p2(4) == 1]
  no_ball_kick -> P6_kick [order 6] : [p6(4) == 1]
  P2_kick -> no_ball_kick : [p2(4) == 0]
  P6_kick -> no_ball_kick : [p6(4) == 0]
  P3_kick -> no_ball_kick : [p3(4) == 0]
  P7_kick -> no_ball_kick : [p7(4) == 0]
  no_ball_kick -> P7_kick [order 7] : [p7(4) == 1]
  no_ball_kick -> P3_kick [order 3] : [p3(4) == 1]
  no_ball_kick -> P8_kick [order 8] : [p8(4) == 1]
  no_ball_kick -> P4_kick [order 4] : [p4(4) == 1]
  P4_kick -> no_ball_kick : [p4(4) == 0]
  P8_kick -> no_ball_kick : [p8(4) == 0]
  data: p1 input; p2 input; p3 input; p4 input; p5 input; p6 input; p7 input; p8 input; KF output

== stateflow chart Control_try_final_2020b/Team_1_behaviour/T1R1(Goal_Keeper)/min_Distance_Finder/R4_O_dist_val/Chart ==
  state calculate
    en:
    dist = 0;
    pos_x = 0;
    pos_y =0;
    dist_x =0;
    dist_y = 0;
    i=0;
    du:
    dist = 0;
    for i=1:7
    if (sen_1_val(i,3) > 4)
    pos_x = R_1_loc(1) + sen_1_val(i,1);
    pos_y = R_1_loc(2) + sen_1_val(i,2);
    dist_x = R_2_loc(1) - pos_x;
    dist_y = R_2_loc(2) - pos_y;
    dist = dist + sqrt((dist_x*dist_x) + (dist_y*dist_y));
    end
    end
  (default) -> calculate
  data: R_1_loc input; sen_1_val input; dist output; R_2_loc input; dist_y local; i local; pos_x local; pos_y local; dist_x local

== matlab function Control_try_final_2020b/Team_1_behaviour/T1R1(Goal_Keeper)/min_Distance_Finder/zero_padding ==
  data: u input; y output
function y = pad(u)
% Zero-pads object detections to work with arrays of buses

y = zeros(7,3);
numElems = min(size(u,1),7);
for idx = 1:numElems
   y(idx,1:3) = u(idx,1:3); 
end
end

== stateflow chart Control_try_final_2020b/Enviornment/Chart ==
  state Vector_combination
    du:
    bot_loc = [R1T1,R2T1,R3T1,R4T1,R1T2,R2T2,R3T2,R4T2]
    bot_vel = [RV1(1),RV2(1),RV3(1),RV4(1),RV5(1),RV6(1),RV7(1),RV8(1)]
  (default) -> Vector_combination
  data: RV1 input; RV2 input; RV3 input; RV4 input; RV7 input; RV5 input; RV6 input; RV8 input; R1T2 input; R2T2 input; R3T2 input; R4T2 input; R4T1 input; R3T1 input; R2T1 input; R1T1 input; bot_loc output; bot_vel output

== stateflow chart Control_try_final_2020b/Team_2_Behaviour/T3_R4(Attacker 2)/Team 1 Behaviour1/Chart3 ==
  state second_coordinate
    du:
    actual_angle = -pi +angle + angle_bot;
  state first_coordinate
    du:
    actual_angle = angle_bot - angle;
  state ffourth_coordinate
    du:
    actual_angle = -(2*pi) + angle + angle_bot
  state Third_coordinate
    du:
    actual_angle =-(pi) - angle + angle_bot;
  (default) -> first_coordinate
  first_coordinate -> second_coordinate [order 1] : [ Rx>Bx && Ry<By ]
  second_coordinate -> first_coordinate [order 1] : [ Rx<Bx && Ry<By]
  ffourth_coordinate -> second_coordinate [order 1] : [ Rx>Bx && Ry<By ]
  first_coordinate -> Third_coordinate [order 3] : [ Rx>Bx && Ry>By]
  second_coordinate -> Third_coordinate [order 3] : [ Rx>Bx && Ry>By ]
  Third_coordinate -> second_coordinate [order 1] : [ Rx>Bx && Ry<By ]
  second_coordinate -> ffourth_coordinate [order 2] : [ Rx<Bx && Ry>By ]
  Third_coordinate -> first_coordinate [order 2] : [ Rx<Bx && Ry<By ]
  ffourth_coordinate -> first_coordinate [order 2] : [ Rx<Bx && Ry<By ]
  first_coordinate -> ffourth_coordinate [order 2] : [ Rx<Bx && Ry>By ]
  Third_coordinate -> ffourth_coordinate [order 3] : [ Rx<Bx && Ry>By ]
  ffourth_coordinate -> Third_coordinate [order 3] : [ Rx>Bx && Ry>By]
  data: Bx input; By input; Rx input; Ry input; angle input; actual_angle output; angle_bot input

== stateflow chart Control_try_final_2020b/Team_2_Behaviour/T3_R4(Attacker 2)/Team 1 Behaviour1/Chart5 ==
  state go_to_ball
    du:
    kick = 0;
    pass_beh = 0;
    if(distance_to_ball < 0.25)
    pass_beh = pass_behaviour_controller(distance_to_goal,nearest_op,nearest_team);
    i = 0;
    else
    velocity = 0.44;
    end
  state avoid
    velocity = -0.44;
  state pass
    du:
    velocity = 0;
    kick = 1;
  state shoot
    du:
    velocity = 0;
    kick = 1;
  state dribble
    du:
    velocity = 0;
    kick = 1;
  (default) -> go_to_ball
  go_to_ball -> avoid [order 4] : [nearest_rob < 0.3 && nearest_rob < 0 ]
  avoid -> go_to_ball : [nearest_rob > 1 || nearest_rob == 0]
  go_to_ball -> pass [order 1] : [pass_beh == 1&& distance_to_ball < 0.25 ]
  dribble -> go_to_ball : [kick == 1]
  go_to_ball -> dribble [order 3] : [pass_beh == 2 && distance_to_ball < 0.25 ]
  pass -> go_to_ball : [kick == 1]
  go_to_ball -> shoot [order 2] : [pass_beh == 3 && distance_to_ball < 0.25 ]
  shoot -> go_to_ball : [kick == 1]
  data: distancetogoal function_input; nearest_oponent_distance function_input; nearest_team_player_distance function_input; pass_behaviour function_output; kick output =0; distance_to_ball input; velocity output; nearest_team input; nearest_op input; distance_to_goal input; pass_beh output =0; i local =1; nearest_rob input
  function pass_behaviour  = pass_behaviour_controller(distancetogoal,nearest_oponent_distance,nearest_team_player_distance):
    | function pass_behaviour  = pass_behaviour_controller(distancetogoal,nearest_oponent_distance,nearest_team_player_distance)
    | %PASS_BEHAVIOR Summary of this function goes here
    | %   Detailed explanation goes here
    | behaviourFuzzyFile= getFISCodeGenerationData('pass_behaviour.fis');
    | b = evalfis(behaviourFuzzyFile,[distancetogoal,nearest_oponent_distance,nearest_team_player_distance]);
    | 
    | if ( b<0.4 )
    | pass_behaviour=1;
    | elseif ( 0.4<=b && b<0.6 )
    | pass_behaviour=2;
    | else
    | pass_behaviour=3;
    | end
    | 
    | end

== stateflow chart Control_try_final_2020b/Team_2_Behaviour/T3_R4(Attacker 2)/Team 1 Behaviour1/Chart6 ==
  state stop
    du:
    w = 0;
    v=0.25 * velocity;
  state RCW
    du:
    w = -1*1;
    v=0;
  state RCCW
    du:
    w =1*1;
    v=0;
  (default) -> stop
  stop -> RCCW [order 2] : [after(1,sec) && DT > 0]
  stop -> RCW [order 1] : [after(1,sec) && DT < 0]
  RCW -> stop [order 1] : [DT<= 0.1 && DT>= -0.1]
  RCCW -> stop [order 1] : [DT<= 0.1 && DT>= -0.1]
  RCCW -> RCW [order 2] : [DT>0]
  RCW -> RCCW [order 2] : [DT<0]
  data: velocity input; v output; DT input; w output

== matlab function Control_try_final_2020b/Team_2_Behaviour/T3_R4(Attacker 2)/Team 1 Behaviour1/MATLAB Function5 ==
  data: F input; dF output; dis input; dT input
function dF = fcn(F,dis,dT)


F_x_max = max(abs(F(:,1))) ;
% F_y_max = max(abs(F(:,2))) ;

Fmax = sqrt((F_x_max^2)) ;

fc = sqrt(2*dis*dis*dT) ;

if fc <= Fmax
    dF = fc ;
else
    dF = Fmax ;
end

end

== stateflow chart Control_try_final_2020b/Team_1_behaviour/T1R3 (Defender 2)/Team 1 Behaviour1/Chart2 ==
  state go_to_ball
    du:
    kick = 0;
    pass_beh = 0;
    if(distance_to_ball < 0.25)
    pass_beh = pass_behaviour_controller(distance_to_goal,nearest_op,nearest_team);
    i = 0;
    else
    velocity = 0.44;
    end
  state pass
    du:
    velocity = 0;
    kick = 1;
  state shoot
    du:
    velocity = 0;
    kick = 1;
  state dribble
    du:
    velocity = 0;
    kick = 1;
  (default) -> go_to_ball
  go_to_ball -> pass [order 1] : [pass_beh == 1&& distance_to_ball < 0.25 ]
  dribble -> go_to_ball : [kick == 1]
  go_to_ball -> dribble [order 3] : [pass_beh == 2 && distance_to_ball < 0.25 ]
  pass -> go_to_ball : [kick == 1]
  go_to_ball -> shoot [order 2] : [pass_beh == 3 && distance_to_ball < 0.25 ]
  shoot -> go_to_ball : [kick == 1]
  data: distancetogoal function_input; nearest_oponent_distance function_input; nearest_team_player_distance function_input; pass_behaviour function_output; kick output =0; distance_to_ball input; velocity output; nearest_team input; nearest_op input; distance_to_goal input; pass_beh output =0; i local =1
  function pass_behaviour  = pass_behaviour_controller(distancetogoal,nearest_oponent_distance,nearest_team_player_distance):
    | function pass_behaviour  = pass_behaviour_controller(distancetogoal,nearest_oponent_distance,nearest_team_player_distance)
    | %PASS_BEHAVIOR Summary of this function goes here
    | %   Detailed explanation goes here
    | behaviourFuzzyFile= getFISCodeGenerationData('pass_behaviour.fis');
    | b = evalfis(behaviourFuzzyFile,[distancetogoal,nearest_oponent_distance,nearest_team_player_distance]);
    | 
    | if ( b<0.4 )
    | pass_behaviour=1;
    | elseif ( 0.4<=b && b<0.6 )
    | pass_behaviour=2;
    | else
    | pass_behaviour=3;
    | end
    | 
    | end

== stateflow chart Control_try_final_2020b/Team_1_behaviour/T1R3 (defender 1)/Team 1 Behaviour/Chart ==
  state second_coordinate
    du:
    actual_angle = -pi +angle + angle_bot;
  state first_coordinate
    du:
    actual_angle = angle_bot - angle;
  state ffourth_coordinate
    du:
    actual_angle = -(2*pi) + angle + angle_bot
  state Third_coordinate
    du:
    actual_angle =-(pi) - angle + angle_bot;
  (default) -> first_coordinate
  first_coordinate -> second_coordinate [order 1] : [ Rx>Bx && Ry<By ]
  second_coordinate -> first_coordinate [order 1] : [ Rx<Bx && Ry<By]
  ffourth_coordinate -> second_coordinate [order 1] : [ Rx>Bx && Ry<By ]
  first_coordinate -> Third_coordinate [order 3] : [ Rx>Bx && Ry>By]
  second_coordinate -> Third_coordinate [order 3] : [ Rx>Bx && Ry>By ]
  Third_coordinate -> second_coordinate [order 1] : [ Rx>Bx && Ry<By ]
  second_coordinate -> ffourth_coordinate [order 2] : [ Rx<Bx && Ry>By ]
  Third_coordinate -> first_coordinate [order 2] : [ Rx<Bx && Ry<By ]
  ffourth_coordinate -> first_coordinate [order 2] : [ Rx<Bx && Ry<By ]
  first_coordinate -> ffourth_coordinate [order 2] : [ Rx<Bx && Ry>By ]
  Third_coordinate -> ffourth_coordinate [order 3] : [ Rx<Bx && Ry>By ]
  ffourth_coordinate -> Third_coordinate [order 3] : [ Rx>Bx && Ry>By]
  data: Bx input; By input; Rx input; Ry input; angle input; actual_angle output; angle_bot input

== stateflow chart Control_try_final_2020b/Team_1_behaviour/T1R3 (defender 1)/Team 1 Behaviour/Chart3 ==
  state stop
    du:
    w = 0;
    v=0.25 * velocity;
  state RCW
    du:
    w = -1*1;
    v=0;
  state RCCW
    du:
    w =1*1;
    v=0;
  (default) -> stop
  stop -> RCCW [order 2] : [after(1,sec) && DT > 0]
  stop -> RCW [order 1] : [after(1,sec) && DT < 0]
  RCW -> stop [order 1] : [DT<= 0.1 && DT>= -0.1]
  RCCW -> stop [order 1] : [DT<= 0.1 && DT>= -0.1]
  RCCW -> RCW [order 2] : [DT>0]
  RCW -> RCCW [order 2] : [DT<0]
  data: velocity input; v output; DT input; w output
